simulink model "diagrama2d"  (Simulink 5.0)
settings: Solver=ode45  StartTime=0.0  StopTime=500  RelTol=1e-3
undefined symbols (not defined in the file): ts
libraries: simulink x15, dsparch4 x3, dspstat3 x2, dsparch3 x1, dspmtrx3 x1, dspsigops x1
settings Model: LastModifiedBy=pc1

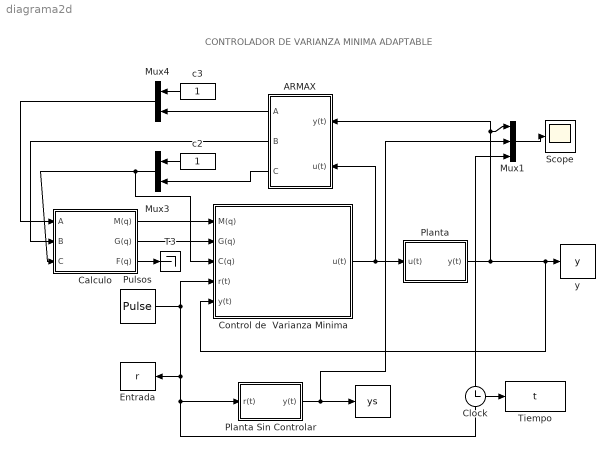
== system diagrama2d ==
  note: CONTROLADOR DE VARIANZA MINIMA ADAPTABLE
  "  " : ToWorkspace  VariableName=ys  SampleTime=ts  SaveFormat=Array
  ARMAX : Subsystem  Orientation=left
  Calculo : Subsystem  mask{na=3, nc=3, nk=0}
  Clock : Clock
      settings: Decimation=10
  Control de  Varianza Minima : Subsystem  Priority=347866248
      settings: ErrorFcn=Control
      mask Type: CONTROL
      mask Display: disp('Controlador')
  Entrada : ToWorkspace  VariableName=r  SampleTime=ts  SaveFormat=Array
  Mux1 : Mux  Inputs=3
  Mux3 : Mux  Orientation=left  Inputs=2
  Mux4 : Mux  Orientation=left  Inputs=2
  Planta : Subsystem
  Planta Sin Controlar : Subsystem
  Pulsos : DiscretePulseGenerator  PulseType=Time based  Amplitude=2  Period=20  PulseWidth=50
  Scope : Scope
  T3 : Terminator
  Tiempo : ToWorkspace  VariableName=t  SampleTime=ts  SaveFormat=Array
  c2 : Constant  Orientation=left
  c3 : Constant  Orientation=left
  y : ToWorkspace  VariableName=y  SampleTime=ts  SaveFormat=Array
  wires:
  Clock/1 -> Tiempo/1
  Control de  Varianza Minima/1(u(t)) -> Planta/1(u(t)), ARMAX/2(u(t))
  Planta/1(y(t)) -> y/1, Control de  Varianza Minima/5(y(t)), ARMAX/1(y(t)), Mux1/1
  Pulsos/1 -> Control de  Varianza Minima/4(r(t)), Entrada/1, Planta Sin Controlar/1(r(t)), Mux1/3
  Planta Sin Controlar/1(y(t)) -> "  "/1, Mux1/2
  Calculo/3(F(q)) -> T3/1
  c2/1 -> Mux3/1
  ARMAX/3(C) -> Mux3/2
  Mux3/1 -> Calculo/3(C), Control de  Varianza Minima/3(C(q))
  c3/1 -> Mux4/1
  ARMAX/1(A) -> Mux4/2
  Mux4/1 -> Calculo/1(A)
  ARMAX/2(B) -> Calculo/2(B)
  Calculo/2(G(q)) -> Control de  Varianza Minima/2(G(q))
  Calculo/1(M(q)) -> Control de  Varianza Minima/1(M(q))
  Mux1/1 -> Scope/1

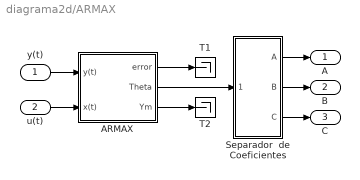
== system diagrama2d/ARMAX ==
  y(t) : Inport
  u(t) : Inport  Port=2
  ARMAX : Subsystem  mask{L=0.991, ts=.1, nk=0, na=3, nb=2, nc=3}
      mask prompts: L "valor landa"; ts "valor ts"; nk "valor nk"; na "Valor na"; nb "valor nb"; nc "valor nc"
  Separador  de Coeficientes : Subsystem  mask{na=3, nb=2, nc=3, ts=0.1}
      mask prompts: ts "Tiempo de Muestreo"
  T1 : Terminator
  T2 : Terminator
  A : Outport
  B : Outport  Port=2
  C : Outport  Port=3
  wires:
  Separador  de Coeficientes/3(C) -> C/1
  Separador  de Coeficientes/2(B) -> B/1
  Separador  de Coeficientes/1(A) -> A/1
  u(t)/1 -> ARMAX/2(x(t))
  y(t)/1 -> ARMAX/1(y(t))
  ARMAX/3(Ym) -> T2/1
  ARMAX/1(error) -> T1/1
  ARMAX/2(Theta) -> Separador  de Coeficientes/1(theta)

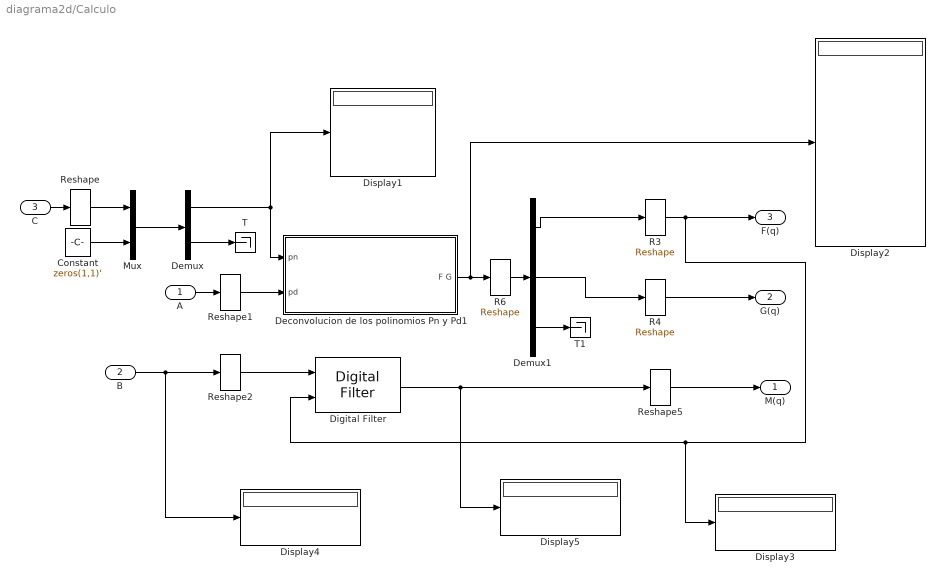
== system diagrama2d/Calculo ==
  A : Inport
  B : Inport  Port=2
  C : Inport  Port=3
  Constant : Constant  Value=zeros(1,1)'
  Deconvolucion de los polinomios Pn y Pd1 : Subsystem  AncestorBlock=Blockset_Practica2/Deconvolucion de los polinomios Pn y Pd1
      mask Display: disp('Division de los\n  polinomios pn y pd\n  \n [F,G] = deconv (pn,pd)')
  Demux : Demux  Outputs=[4 1]
  Demux1 : Demux  Outputs=[1 4 5]
  Digital Filter : dsparch4/Digital Filter  TypePopup=FIR (all zeros)  IIRFiltStruct=Direct form II transposed  AllPoleFiltStruct=Direct form  FIRFiltStruct=Direct form  CoeffSource=Input port(s)  NumCoeffs=[1 2]  DenCoeffs=[1 0.1]  BiQuadCoeffs=[1 0.3 0.4 1 0.1 0.2]  LatticeCoeffs=[0.2 0.4]  denIgnore=on  FiltPerSampPopup=One filter per sample  IC=0  ICnum=0  ICden=0
  Display{1..5} (5 alike) : Display
  Mux : Mux  Inputs=2
  R3 : simulink/Math Operations/Reshape  OutputDimensionality=Column vector  OutputDimensions=[1,1]
  R4 : simulink/Math Operations/Reshape  OutputDimensionality=Column vector  OutputDimensions=[1,1]
  R6 : simulink/Math Operations/Reshape  OutputDimensionality=Column vector  OutputDimensions=[1,1]
  Reshape{,1..2,5} (4 alike) : simulink/Math Operations/Reshape  OutputDimensionality=Column vector  OutputDimensions=[1,1]
  T : Terminator
  T1 : Terminator
  M(q) : Outport
  G(q) : Outport  Port=2
  F(q) : Outport  Port=3
  wires:
  A/1 -> Reshape1/1
  Constant/1 -> Mux/2
  C/1 -> Reshape/1
  Mux/1 -> Demux/1
  Demux/1 -> Deconvolucion de los polinomios Pn y Pd1/1(pn), Display1/1
  Demux/2 -> T/1
  Reshape/1 -> Mux/1
  Reshape1/1 -> Deconvolucion de los polinomios Pn y Pd1/2(pd)
  Deconvolucion de los polinomios Pn y Pd1/1(F G) -> R6/1, Display2/1
  Demux1/1 -> R3/1
  B/1 -> Reshape2/1, Display4/1
  Digital Filter/1 -> Reshape5/1, Display5/1
  Reshape2/1 -> Digital Filter/1
  R3/1 -> F(q)/1, Digital Filter/2, Display3/1
  R4/1 -> G(q)/1
  Reshape5/1 -> M(q)/1
  R6/1 -> Demux1/1
  Demux1/3 -> T1/1
  Demux1/2 -> R4/1

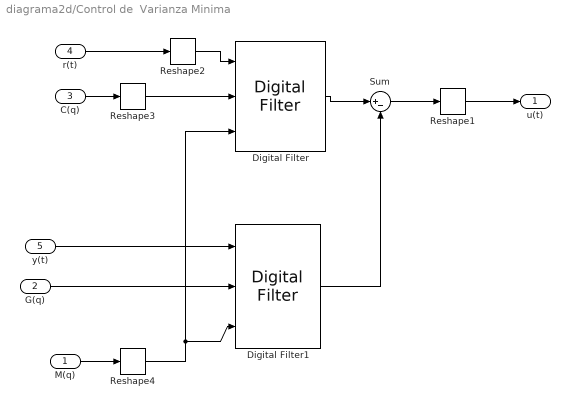
== system diagrama2d/Control de  Varianza Minima ==
  M(q) : Inport
  G(q) : Inport  Port=2
  C(q) : Inport  Port=3
  r(t) : Inport  Port=4
  y(t) : Inport  Port=5
  Digital Filter : dsparch4/Digital Filter  TypePopup=IIR (poles & zeros)  IIRFiltStruct=Direct form II transposed  AllPoleFiltStruct=Direct form  FIRFiltStruct=Direct form  CoeffSource=Input port(s)  NumCoeffs=[1 2]  DenCoeffs=[1 0.1]  BiQuadCoeffs=[1 0.3 0.4 1 0.1 0.2]  LatticeCoeffs=[0.2 0.4]  denIgnore=off  FiltPerSampPopup=One filter per frame  IC=0  ICnum=0  ICden=0
  Digital Filter1 : dsparch4/Digital Filter  TypePopup=IIR (poles & zeros)  IIRFiltStruct=Direct form II transposed  AllPoleFiltStruct=Direct form  FIRFiltStruct=Direct form  CoeffSource=Input port(s)  NumCoeffs=[1 2]  DenCoeffs=[1 0.1]  BiQuadCoeffs=[1 0.3 0.4 1 0.1 0.2]  LatticeCoeffs=[0.2 0.4]  denIgnore=off  FiltPerSampPopup=One filter per frame  IC=0  ICnum=0  ICden=0
  Reshape1 : simulink/Math Operations/Reshape  OutputDimensionality=Customize  OutputDimensions=[1]
  Reshape2 : simulink/Math Operations/Reshape  OutputDimensionality=Customize  OutputDimensions=[1]
  Reshape3 : simulink/Math Operations/Reshape  OutputDimensionality=Column vector  OutputDimensions=[1]
  Reshape4 : simulink/Math Operations/Reshape  OutputDimensionality=Column vector  OutputDimensions=[1]
  Sum : Sum  Inputs=|+-  SaturateOnIntegerOverflow=on
  u(t) : Outport
  wires:
  Sum/1 -> Reshape1/1
  Digital Filter1/1 -> Sum/2
  Digital Filter/1 -> Sum/1
  y(t)/1 -> Digital Filter1/1
  G(q)/1 -> Digital Filter1/2
  C(q)/1 -> Reshape3/1
  r(t)/1 -> Reshape2/1
  Reshape2/1 -> Digital Filter/1
  Reshape1/1 -> u(t)/1
  Reshape3/1 -> Digital Filter/2
  M(q)/1 -> Reshape4/1
  Reshape4/1 -> Digital Filter1/3, Digital Filter/3

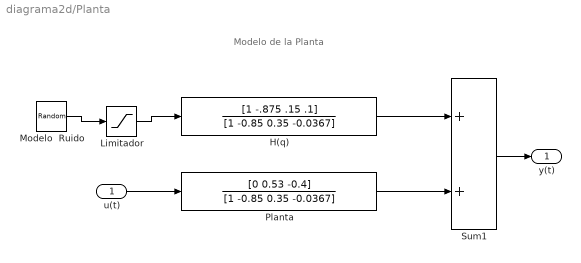
== system diagrama2d/Planta ==
  note: Modelo de la Planta
  u(t) : Inport
  H(q) : DiscreteFilter  Numerator=[1 -.875 .15 .1]  Denominator=[1 -0.85 0.35 -0.0367]  SampleTime=.1
  Limitador : Saturate  UpperLimit=0.005  LowerLimit=-0.005
  Modelo  Ruido : RandomNumber  Variance=0.005  SampleTime=0.1
  Planta : DiscreteFilter  Numerator=[0 0.53 -0.4]  Denominator=[1 -0.85 0.35 -0.0367]  SampleTime=.1
  Sum1 : Sum  SaturateOnIntegerOverflow=on
  y(t) : Outport
  wires:
  Sum1/1 -> y(t)/1
  Planta/1 -> Sum1/2
  u(t)/1 -> Planta/1
  H(q)/1 -> Sum1/1
  Modelo  Ruido/1 -> Limitador/1
  Limitador/1 -> H(q)/1

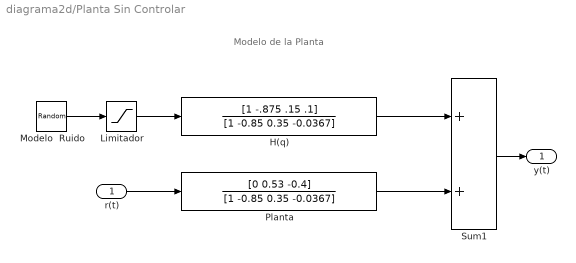
== system diagrama2d/Planta Sin Controlar ==
  note: Modelo de la Planta
  r(t) : Inport
  H(q) : DiscreteFilter  Numerator=[1 -.875 .15 .1]  Denominator=[1 -0.85 0.35 -0.0367]  SampleTime=.1
  Limitador : Saturate  UpperLimit=0.005  LowerLimit=-0.005
  Modelo  Ruido : RandomNumber  Variance=0.005  SampleTime=0.1
  Planta : DiscreteFilter  Numerator=[0 0.53 -0.4]  Denominator=[1 -0.85 0.35 -0.0367]  SampleTime=.1
  Sum1 : Sum  SaturateOnIntegerOverflow=on
  y(t) : Outport
  wires:
  Sum1/1 -> y(t)/1
  Planta/1 -> Sum1/2
  r(t)/1 -> Planta/1
  H(q)/1 -> Sum1/1
  Modelo  Ruido/1 -> Limitador/1
  Limitador/1 -> H(q)/1

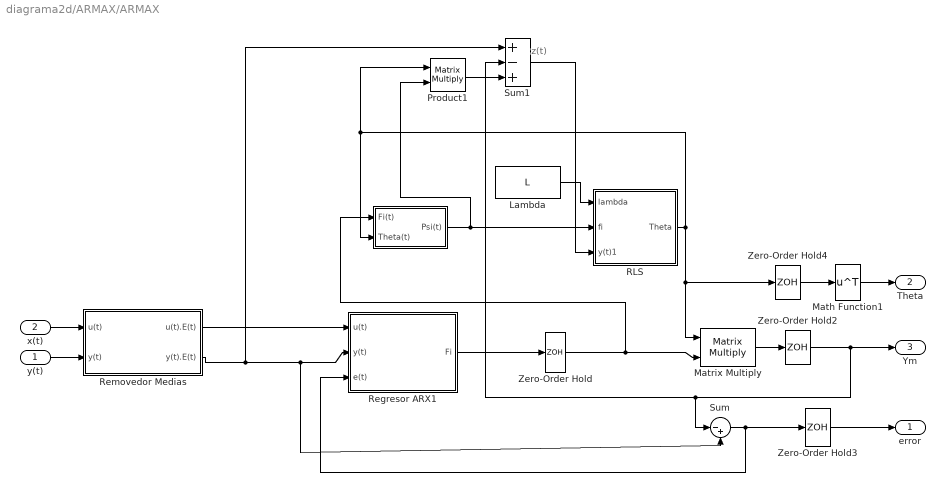
== system diagrama2d/ARMAX/ARMAX ==
  note: z(t)
  y(t) : Inport
  x(t) : Inport  Port=2
  "  " : Subsystem
  Lambda : Constant  Value=L  ShowAdditionalParam=on
  Math Function1 : Math  Operator=transpose
  Matrix Multiply : dspmtrx3/Matrix Multiply  numInputPorts=2  OptimizationLevel=None
  Product1 : Product  Multiplication=Matrix(*)  SaturateOnIntegerOverflow=on  InputSameDT=on
  RLS : Subsystem
  Regresor ARX1 : Subsystem
  Removedor Medias : Subsystem
  Sum : Sum  Inputs=|-+  SaturateOnIntegerOverflow=on  InputSameDT=on
  Sum1 : Sum  Inputs=+-+  SaturateOnIntegerOverflow=on  InputSameDT=on
  Zero-Order Hold{,2..4} (4 alike) : ZeroOrderHold  SampleTime=ts
  error : Outport
  Theta : Outport  Port=2
  Ym : Outport  Port=3
  wires:
  Math Function1/1 -> Theta/1
  Zero-Order Hold4/1 -> Math Function1/1
  RLS/1(Theta) -> Matrix Multiply/1, Zero-Order Hold4/1, "  "/2(Theta(t)), Product1/1
  Lambda/1 -> RLS/1(lambda)
  "  "/1(Psi(t)) -> RLS/2(fi), Product1/2
  Regresor ARX1/1(Fi) -> Zero-Order Hold/1
  Removedor Medias/2(y(t).E(t)) -> Sum/2, Regresor ARX1/2(y(t)), Sum1/1
  Removedor Medias/1(u(t).E(t)) -> Regresor ARX1/1(u(t))
  y(t)/1 -> Removedor Medias/2(y(t))
  x(t)/1 -> Removedor Medias/1(u(t))
  Zero-Order Hold/1 -> Matrix Multiply/2, "  "/1(Fi(t))
  Matrix Multiply/1 -> Zero-Order Hold2/1
  Zero-Order Hold2/1 -> Ym/1, Sum/1, Sum1/2
  Sum/1 -> Regresor ARX1/3(e(t)), Zero-Order Hold3/1
  Zero-Order Hold3/1 -> error/1
  Product1/1 -> Sum1/3
  Sum1/1 -> RLS/3(y(t)1)

== system diagrama2d/ARMAX/Separador  de Coeficientes ==
  theta : Inport  PortDimensions=[na+nb+nc;1]  SampleTime=ts
  Demux : Demux  Outputs=[na,nb,nc]
  A : Outport
  B : Outport  Port=2
  C : Outport  Port=3
  wires:
  Demux/3 -> C/1
  Demux/2 -> B/1
  theta/1 -> Demux/1
  Demux/1 -> A/1

== system diagrama2d/Calculo/Deconvolucion de los polinomios Pn y Pd1 ==
  pn : Inport  SampleTime=.1
  pd : Inport  Port=2
  Mux : Mux
  S-Function : S-Function  FunctionName=deconvolucion
  Width : Width
  Width1 : Width
  F G : Outport
  wires:
  S-Function/1 -> F G/1
  pd/1 -> Mux/4, Width1/1
  pn/1 -> Mux/3, Width/1
  Width1/1 -> Mux/2
  Width/1 -> Mux/1
  Mux/1 -> S-Function/1

== system diagrama2d/ARMAX/ARMAX/   ==
  Fi(t) : Inport
  Theta(t) : Inport  Port=2
  filtro iir : Subsystem
  Psi(t) : Outport
  wires:
  filtro iir/1(Out1) -> Psi(t)/1
  Theta(t)/1 -> filtro iir/2(In2)
  Fi(t)/1 -> filtro iir/1(In1)

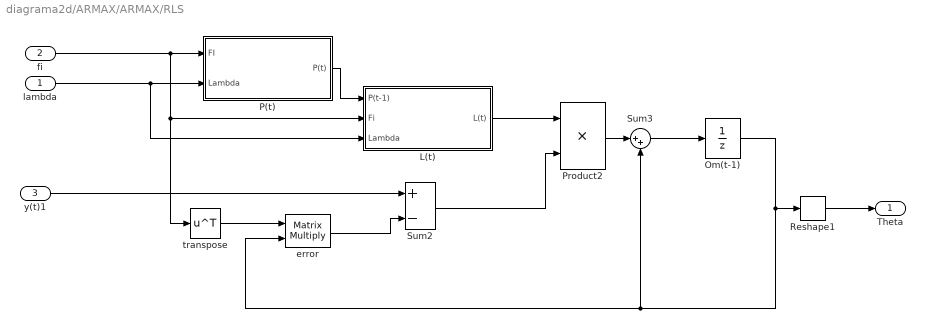
== system diagrama2d/ARMAX/ARMAX/RLS ==
  lambda : Inport
  fi : Inport  Port=2
  y(t)1 : Inport  Port=3
  L(t) : Subsystem
  Om(t-1) : UnitDelay  X0=zeros(1,na+nb+nc)'+.2  SampleTime=ts
  P(t) : Subsystem
  Product2 : Product  SaturateOnIntegerOverflow=on  InputSameDT=on
  Reshape1 : simulink/Math Operations/Reshape  OutputDimensionality=Row vector  OutputDimensions=[1,1]
  Sum2 : Sum  Inputs=+-  SaturateOnIntegerOverflow=on  InputSameDT=on
  Sum3 : Sum  Inputs=|++  SaturateOnIntegerOverflow=on  InputSameDT=on
  error : Product  Multiplication=Matrix(*)  SaturateOnIntegerOverflow=on  InputSameDT=on
  transpose : Math  Operator=transpose
  Theta : Outport
  wires:
  Reshape1/1 -> Theta/1
  lambda/1 -> L(t)/3(Lambda), P(t)/2(Lambda)
  fi/1 -> transpose/1, L(t)/2(Fi), P(t)/1(FI)
  P(t)/1("P(t) ") -> L(t)/1(P(t-1))
  L(t)/1(L(t)) -> Product2/1
  Product2/1 -> Sum3/1
  Sum3/1 -> Om(t-1)/1
  Sum2/1 -> Product2/2
  y(t)1/1 -> Sum2/1
  error/1 -> Sum2/2
  Om(t-1)/1 -> Reshape1/1, error/2, Sum3/2
  transpose/1 -> error/1

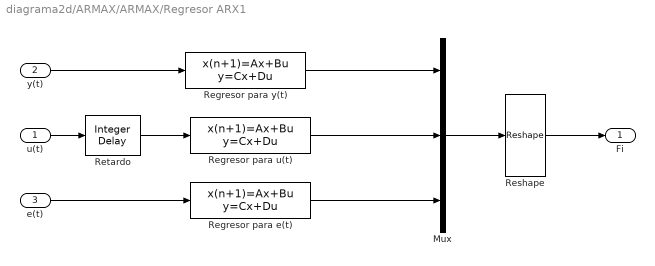
== system diagrama2d/ARMAX/ARMAX/Regresor ARX1 ==
  u(t) : Inport
  y(t) : Inport  Port=2
  e(t) : Inport  Port=3
  Mux : Mux  Inputs=3
  Regresor para e(t) : DiscreteStateSpace  A=[zeros(1,nc);eye(nc-1,nc)]  B=[1,zeros(1,nc-1)]'  C=eye(nc)  D=[zeros(nc,1)]  SampleTime=ts
  Regresor para u(t) : DiscreteStateSpace  A=[zeros(1,nb);eye(nb-1,nb)]  B=[1,zeros(1,nb-1)]'  C=eye(nb)  D=[zeros(nb,1)]  SampleTime=ts
  Regresor para y(t) : DiscreteStateSpace  A=[zeros(1,na);eye(na-1,na)]  B=[-1,zeros(1,na-1)]'  C=eye(na)  D=[zeros(na,1)]  SampleTime=ts
  Reshape : simulink/Math Operations/Reshape  OutputDimensionality=Column vector  OutputDimensions=[1,1]
  Retardo : dspsigops/Integer Delay  delay=nk  ic=0  reset_popup=None
  Fi : Outport
  wires:
  Regresor para e(t)/1 -> Mux/3
  Reshape/1 -> Fi/1
  Regresor para y(t)/1 -> Mux/1
  Regresor para u(t)/1 -> Mux/2
  y(t)/1 -> Regresor para y(t)/1
  Mux/1 -> Reshape/1
  u(t)/1 -> Retardo/1
  Retardo/1 -> Regresor para u(t)/1
  e(t)/1 -> Regresor para e(t)/1

== system diagrama2d/ARMAX/ARMAX/Removedor Medias ==
  u(t) : Inport
  y(t) : Inport  Port=2
  Romovedor de  valores medios : Subsystem
  Romovedor de  valores medios1 : Subsystem
  u(t).E(t) : Outport
  y(t).E(t) : Outport  Port=2
  wires:
  Romovedor de  valores medios1/1(y(t)-Ex(t)) -> y(t).E(t)/1
  y(t)/1 -> Romovedor de  valores medios1/1(y(t))
  Romovedor de  valores medios/1(x(t)-Ex(t)) -> u(t).E(t)/1
  u(t)/1 -> Romovedor de  valores medios/1(x(t))

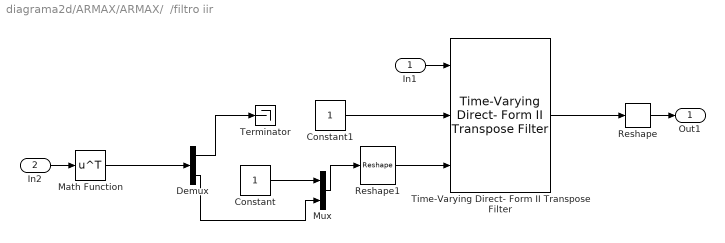
== system diagrama2d/ARMAX/ARMAX/  /filtro iir ==
  In1 : Inport
  In2 : Inport  Port=2
  Constant : Constant
  Constant1 : Constant
  Demux : Demux  Outputs=[na+nb,nc]
  Math Function : Math  Operator=transpose
  Mux : Mux  Inputs=2
  Reshape : simulink/Math Operations/Reshape  OutputDimensionality=Column vector  OutputDimensions=[1,1]
  Reshape1 : simulink/Math Operations/Reshape  OutputDimensionality=Column vector  OutputDimensions=[1,1]
  Terminator : Terminator
  Time-Varying Direct- Form II Transpose Filter : dsparch3/Time-Varying Direct- Form II Transpose Filter  NumDen=Pole-Zero (IIR)  ic=0  filtCheck=on  FiltPerFrame=One Filter Per Frame Time
  Out1 : Outport
  wires:
  In2/1 -> Math Function/1
  Reshape/1 -> Out1/1
  In1/1 -> Time-Varying Direct- Form II Transpose Filter/1
  Reshape1/1 -> Time-Varying Direct- Form II Transpose Filter/3
  Mux/1 -> Reshape1/1
  Math Function/1 -> Demux/1
  Demux/2 -> Mux/2
  Constant/1 -> Mux/1
  Constant1/1 -> Time-Varying Direct- Form II Transpose Filter/2
  Demux/1 -> Terminator/1
  Time-Varying Direct- Form II Transpose Filter/1 -> Reshape/1

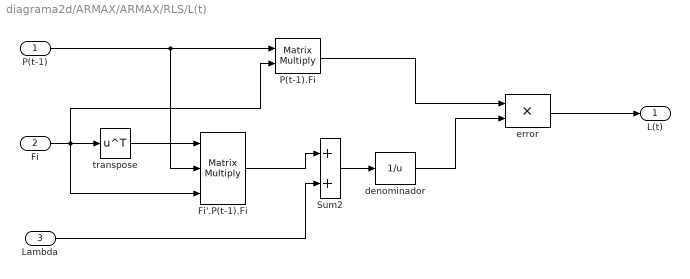
== system diagrama2d/ARMAX/ARMAX/RLS/L(t) ==
  P(t-1) : Inport
  Fi : Inport  Port=2
  Lambda : Inport  Port=3
  Fi'.P(t-1).Fi : Product  Inputs=3  Multiplication=Matrix(*)  SaturateOnIntegerOverflow=on  InputSameDT=on
  P(t-1).Fi : Product  Multiplication=Matrix(*)  ShowAdditionalParam=on  SaturateOnIntegerOverflow=on  InputSameDT=on
  Sum2 : Sum  ShowAdditionalParam=on  SaturateOnIntegerOverflow=on  InputSameDT=on
  denominador : Fcn  Expr=1/u
  error : Product  SaturateOnIntegerOverflow=on  InputSameDT=on
  transpose : Math  Operator=transpose
  L(t) : Outport
  wires:
  Lambda/1 -> Sum2/2
  Fi'.P(t-1).Fi/1 -> Sum2/1
  error/1 -> L(t)/1
  P(t-1)/1 -> P(t-1).Fi/1, Fi'.P(t-1).Fi/2
  P(t-1).Fi/1 -> error/1
  denominador/1 -> error/2
  Sum2/1 -> denominador/1
  transpose/1 -> Fi'.P(t-1).Fi/1
  Fi/1 -> Fi'.P(t-1).Fi/3, transpose/1, P(t-1).Fi/2

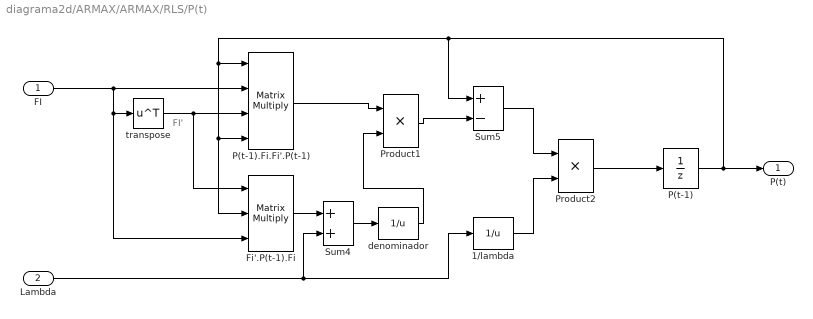
== system diagrama2d/ARMAX/ARMAX/RLS/P(t) ==
  note: FI'
  FI : Inport
  Lambda : Inport  Port=2
  1/lambda : Fcn  Expr=1/u
  Fi'.P(t-1).Fi : Product  Inputs=3  Multiplication=Matrix(*)  SaturateOnIntegerOverflow=on  InputSameDT=on
  P(t-1) : UnitDelay  X0=100000*eye(na+nb+nc)  SampleTime=ts
  P(t-1).Fi.Fi'.P(t-1) : Product  Inputs=4  Multiplication=Matrix(*)  SaturateOnIntegerOverflow=on  InputSameDT=on
  Product1 : Product  SaturateOnIntegerOverflow=on  InputSameDT=on
  Product2 : Product  SaturateOnIntegerOverflow=on  InputSameDT=on
  Sum4 : Sum  SaturateOnIntegerOverflow=on  InputSameDT=on
  Sum5 : Sum  Inputs=+-  SaturateOnIntegerOverflow=on  InputSameDT=on
  denominador : Fcn  Expr=1/u
  transpose : Math  Operator=transpose
  "P(t) " : Outport
  wires:
  denominador/1 -> Product1/2
  1/lambda/1 -> Product2/2
  Sum5/1 -> Product2/1
  Product1/1 -> Sum5/2
  P(t-1).Fi.Fi'.P(t-1)/1 -> Product1/1
  Sum4/1 -> denominador/1
  Fi'.P(t-1).Fi/1 -> Sum4/1
  P(t-1)/1 -> "P(t) "/1, Fi'.P(t-1).Fi/2, P(t-1).Fi.Fi'.P(t-1)/4, P(t-1).Fi.Fi'.P(t-1)/1, Sum5/1
  Product2/1 -> P(t-1)/1
  Lambda/1 -> Sum4/2, 1/lambda/1
  transpose/1 -> Fi'.P(t-1).Fi/1, P(t-1).Fi.Fi'.P(t-1)/3
  FI/1 -> P(t-1).Fi.Fi'.P(t-1)/2, transpose/1, Fi'.P(t-1).Fi/3

== system diagrama2d/ARMAX/ARMAX/Removedor Medias/Romovedor de  valores medios ==
  x(t) : Inport
  Mean : dspstat3/Mean  run=on  reset_popup=None
  Sum : Sum  Inputs=|-+  SaturateOnIntegerOverflow=on  InputSameDT=on
  Zero-Order Hold : ZeroOrderHold  SampleTime=ts
  x(t)-Ex(t) : Outport
  wires:
  Sum/1 -> x(t)-Ex(t)/1
  Mean/1 -> Sum/1
  Zero-Order Hold/1 -> Sum/2, Mean/1
  x(t)/1 -> Zero-Order Hold/1

== system diagrama2d/ARMAX/ARMAX/Removedor Medias/Romovedor de  valores medios1 ==
  y(t) : Inport
  Mean : dspstat3/Mean  run=on  reset_popup=None
  Sum : Sum  Inputs=|-+  SaturateOnIntegerOverflow=on  InputSameDT=on
  Zero-Order Hold : ZeroOrderHold  SampleTime=ts
  y(t)-Ex(t) : Outport
  wires:
  Sum/1 -> y(t)-Ex(t)/1
  Mean/1 -> Sum/1
  Zero-Order Hold/1 -> Sum/2, Mean/1
  y(t)/1 -> Zero-Order Hold/1
